simulink model "untitled2"  (R2023b)
settings: Solver=VariableStepAuto  StartTime=0.0  StopTime=10.0  RelTol=1e-3
libraries: dspfdesign x3
settings Model: Creator=mrabd  LastModifiedBy=mrabd

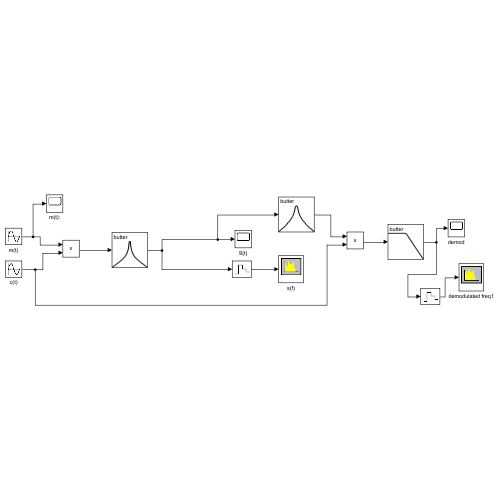
[thumbnail: Simulink's stored preview of the top-level diagram]
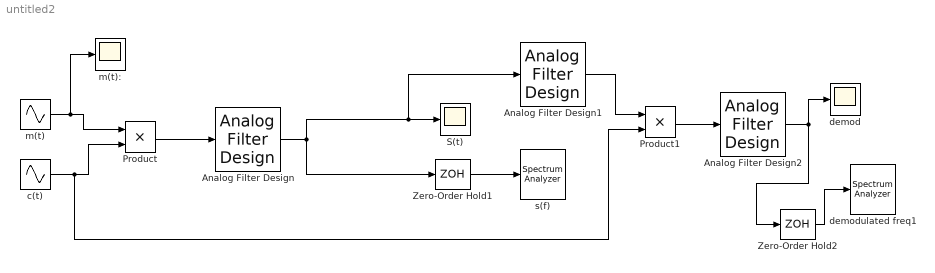
== system untitled2 ==
  Analog Filter Design : dspfdesign/Analog Filter Design  method=Butterworth  filttype=Bandpass  N=8  Wlo=14000  Whi=15000  Rp=2  Rs=40
  Analog Filter Design1 : dspfdesign/Analog Filter Design  method=Butterworth  filttype=Bandpass  N=8  Wlo=13000  Whi=16000  Rp=2  Rs=40
  Analog Filter Design2 : dspfdesign/Analog Filter Design  method=Butterworth  filttype=Lowpass  N=8  Wlo=30000  Whi=15000  Rp=2  Rs=40
  Product : Product
  Product1 : Product
  S(t) : Scope
  Zero-Order Hold1 : ZeroOrderHold  SampleTime=-1
  Zero-Order Hold2 : ZeroOrderHold  SampleTime=-1
  c(t) : Sin  Frequency=15000  SampleTime=0
  demod : Scope
  demodulated freq1 : SpectrumAnalyzer  WindowPosition=[770.000000,42.000000,766.000000,793.000000,]  Visible=on  ScopeFrameLocation=window  SampleRateSource=Property  SampleRate=44.1e3  PlotAsTwoSidedSpectrum=off  FrequencyScale=Log  FrequencySpan=Start and stop frequencies  StartFrequency=20  StopFrequency=20e3  FilterSharpness=0.5  YLimits=[-163.18965215,29.58400153]  SelectedToolstripTab=spectrumAnalyzerToolstrip.measurementsTab
  m(t) : Sin  Amplitude=0.85  Frequency=1000  SampleTime=0
  m(t): : Scope
  s(f) : SpectrumAnalyzer  WindowPosition=[2.000000,42.000000,766.000000,793.000000,]  Visible=on  ScopeFrameLocation=window  SampleRateSource=Property  SampleRate=44.1e3  PlotAsTwoSidedSpectrum=off  FrequencyScale=Log  FrequencySpan=Start and stop frequencies  StartFrequency=20  StopFrequency=20e3  FilterSharpness=0.5  YLimits=[-203.14916758,39.04823033]  SelectedToolstripTab=spectrumAnalyzerToolstrip.measurementsTab
  wires:
  m(t)/1 -> m(t):/1, Product/1
  c(t)/1 -> Product1/2, Product/2
  Product/1 -> Analog Filter Design/1
  Analog Filter Design/1 -> Analog Filter Design1/1, S(t)/1, Zero-Order Hold1/1
  Zero-Order Hold1/1 -> s(f)/1
  Analog Filter Design1/1 -> Product1/1
  Product1/1 -> Analog Filter Design2/1
  Analog Filter Design2/1 -> demod/1, Zero-Order Hold2/1
  Zero-Order Hold2/1 -> demodulated freq1/1
